simulink model "Alireza_Abassi"  (R2021a)
settings: Solver=FixedStepAuto  StartTime=0.0  StopTime=10  FixedStep=0.01  RelTol=1e-3
values from neighbouring files (symbols this model uses):
  A = [0,             0,          1,          0 ... (first row only)    [MyTask.m]
  B = [0 ... (first row only)    [MyTask.m]
  C = [0,  1,  0,  0;]    [MyTask.m]
  D = 0    [MyTask.m]
undefined symbols (not defined in the file or in its folder): den, k2, num
libraries: slctrlblks x1
settings Model: Creator=alire  LastModifiedBy=alire

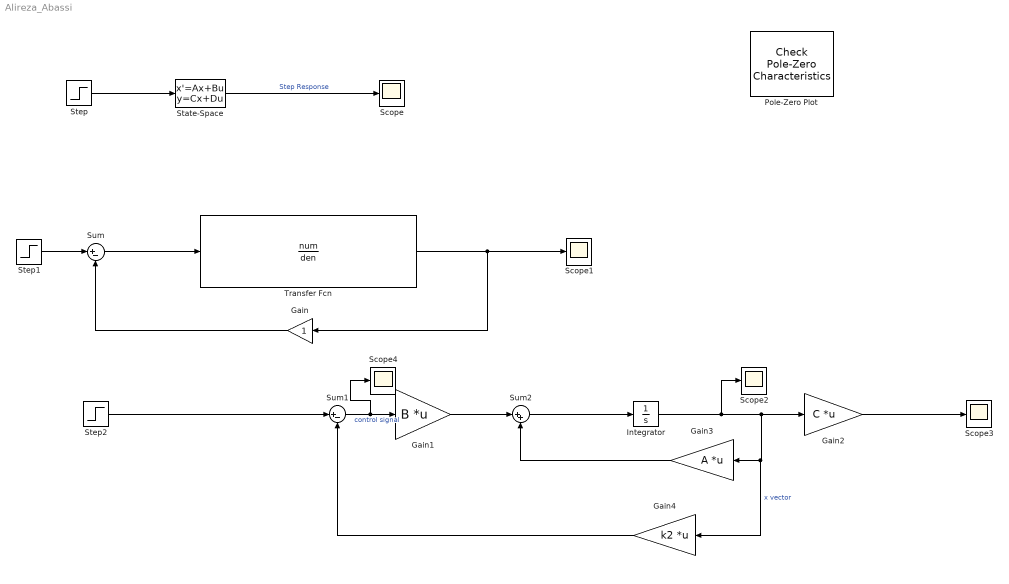
== system Alireza_Abassi ==
  Gain : Gain
  Gain1 : Gain  Gain=B  Multiplication=Matrix(K*u) (u vector)
  Gain2 : Gain  Gain=C  Multiplication=Matrix(K*u) (u vector)
  Gain3 : Gain  Gain=A  Multiplication=Matrix(K*u) (u vector)
  Gain4 : Gain  Gain=k2  Multiplication=Matrix(K*u) (u vector)
  Integrator : Integrator
  Pole-Zero Plot : slctrlblks/Model Verification/Check Pole-Zero Characteristics  InstantiateOnLoad=on  SaveOperatingPoints=off  LinearizationIOs={'/Step2', 1, 'in', 'off', '';'/Gain2', 1, 'out', 'off', ''}  LinearizeAt=SnapshotTimes  SnapshotTimes=[0]  TriggerType=rising  SampleTime=auto  RateConversionMethod=zoh  PreWarpFreq=10  UseExactDelayModel=off  UseFullBlockNameLabels=off  UseBusSignalLabels=off  enabled=on  stopWhenAssertionFail=off  export=off  ViewDlgPos=[1 49 1536 740.8]  LaunchViewOnOpen=off  OpenViewOnLoad=off  FrequencyUnits=rad/s  MagnitudeUnits=dB  PhaseUnits=deg  TimeUnits=seconds  EnableSettlingTime=off  SettlingTime=[]  EnablePercentOvershoot=off  PercentOvershoot=[]  EnableDampingRatio=off  DampingRatio=[]  EnableNaturalFrequency=off  NaturalFrequencyBound=>=  NaturalFrequency=[]
      settings: SourceProductBaseCode=SD  SaveToWorkspace=off  SaveName=sys
  Scope{,1..4} (5 alike) : Scope
  State-Space : StateSpace  A=A  B=B  C=C  D=D  InitialCondition=0
  Step : Step  SampleTime=0
  Step1 : Step  SampleTime=0
  Step2 : Step  SampleTime=0
  Sum : Sum  Inputs=|+-
  Sum1 : Sum  Inputs=|+-
  Sum2 : Sum  Inputs=|++
  Transfer Fcn : TransferFcn  Numerator=num  Denominator=den
  wires:
  Step/1 -> State-Space/1
  Transfer Fcn/1 -> Gain/1, Scope1/1
  Step1/1 -> Sum/1
  Sum/1 -> Transfer Fcn/1
  Gain/1 -> Sum/2
  Sum1/1 -> Scope4/1, Gain1/1  "control signal"
  Gain1/1 -> Sum2/1
  Sum2/1 -> Integrator/1
  Integrator/1 -> Gain2/1, Gain4/1, Gain3/1, Scope2/1  "x vector"
  Gain3/1 -> Sum2/2
  Gain2/1 -> Scope3/1
  Step2/1 -> Sum1/1
  State-Space/1 -> Scope/1  "Step Response"
  Gain4/1 -> Sum1/2
